simulink model "sampleModel282"  (R2021b)
settings: Solver=VariableStepAuto  StartTime=0.0  StopTime=10.0  RelTol=1e-3
undefined symbols (not defined in the file or in its folder): DiscIntNeverNeededParam, Newton, Raphson
libraries: simulink x13, slpidlib x2
settings Model: Creator=user  LastModifiedBy=user

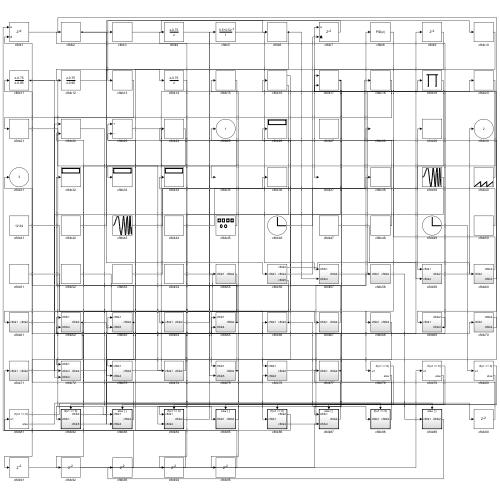
[thumbnail: Simulink's stored preview of the top-level diagram]
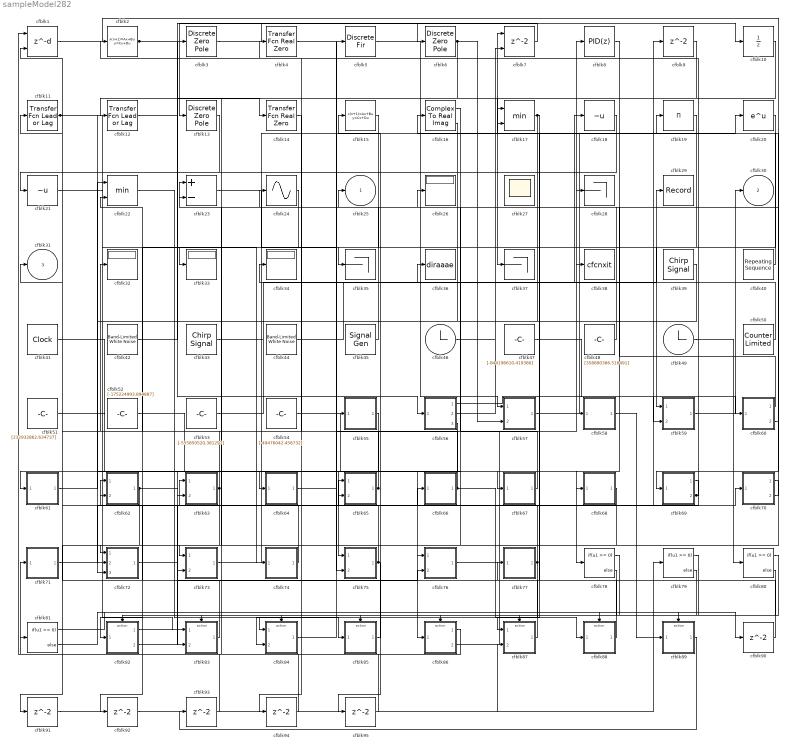
== system sampleModel282 ==
  cfblk1 : Delay  DelayLengthSource=Input port  SampleTime=1
      settings: InputPortMap=u0,p1
  cfblk10 : UnitDelay  HasFrameUpgradeWarning=on
  cfblk11 : simulink/Discrete/Transfer Fcn Lead or Lag  PoleZ=0.95  ZeroZ=0.75  ICPrevOutput=0.0  ICPrevInput=0.0  DoSatur=off
      settings: SourceProductBaseCode=SL
  cfblk12 : simulink/Discrete/Transfer Fcn Lead or Lag  PoleZ=0.95  ZeroZ=0.75  ICPrevOutput=0.0  ICPrevInput=0.0  DoSatur=off
      settings: SourceProductBaseCode=SL
  cfblk13 : DiscreteZeroPole  Poles=[0 0.5]  Gain=1
  cfblk14 : simulink/Discrete/Transfer Fcn Real Zero  ZeroZ=0.75  ICPrevInput=0.0  DoSatur=off
      settings: SourceProductBaseCode=SL
  cfblk15 : DiscreteStateSpace
  cfblk16 : ComplexToRealImag
  cfblk17 : MinMax  Inputs=2
  cfblk18 : UnaryMinus
  cfblk19 : Product  Inputs=*
  cfblk2 : DiscreteStateSpace
  cfblk20 : Math  SaturateOnIntegerOverflow=on
  cfblk21 : UnaryMinus
  cfblk22 : MinMax  Inputs=2
  cfblk23 : Sum  Inputs=+-
  cfblk24 : Sin  TimeSource=Use external signal  SampleTime=0
  cfblk{26,32..34} (4 alike) : Display
  cfblk27 : Scope
      settings: Floating=on
  cfblk28 : Terminator
  cfblk29 : Record  FileSettingsInternal="{\"entries\":[{\"content\":{\"excelSettings\":{\"content\":{},\"type\":\"Streamout.ExcelSettings\"}},\"type\":\"Streamout.FileSettingStorage\",\"uuid\":\"7d52aaf1-a181-40a9-9f35-a4ee466a9437\"}],\"packageUris\":[\"http://schema.mathworks.com/mf0/streamout_blocks/R2020a\"],\"version\":\"1.0\"}"  SignalsInternal="{\"entries\":[{\"content\":{\"signals\":[{\"content\":{\"blockPath\":[\"sampleModel282/cfblk29\"],\"channel\":[],\"dimensions\":[1],\"domain\":\"sampleModel282/cfblk29\",\"lineColor\":\"#fe330a\",\"plots\":[1],\"port\":1,\"sid\":[\"\"],\"signalID\":12055,\"signalName\":\"cfblk44\"},\"type\":\"RecordBlkView.Signal\",\"uuid\":\"b13949a6-b872-4204-8168-bd2ff3b91c96\"}]},\"type\":\"RecordBlkView.InputSignals\",\"uuid\":\"624ad5e0-89e9-4b40-8b6d-38fdad05cf61\"}],\"packageUris\":[\"http://schema.mathworks.com/mf0/streamout_blocks/R2020a\"],\"version\":\"1.0\"}"  VisualizationBindings="{\"sparklinesplugin\":{\"info\":[{\"bindingParametersList\":[],\"subplotID\":1}]}}"
  cfblk3 : DiscreteZeroPole  Poles=[0 0.5]  Gain=1
  cfblk35 : Terminator
  cfblk36 : ToWorkspace  VariableName=diraaae  SaveFormat=Timeseries  SampleTime=-1
  cfblk37 : Terminator
  cfblk38 : ToWorkspace  VariableName=cfcnxit  SaveFormat=Timeseries  SampleTime=-1
  cfblk39 : simulink/Sources/Chirp Signal  f1=[-918796217.277250]  T=[209630549.762623]  f2=[869455804.369112]
  cfblk4 : simulink/Discrete/Transfer Fcn Real Zero  ZeroZ=0.75  ICPrevInput=0.0  DoSatur=off
      settings: SourceProductBaseCode=SL
  cfblk40 : simulink/Sources/Repeating Sequence  rep_seq_t=[0 2]  rep_seq_y=[-594596007.538170, -429150568.442471]
  cfblk41 : DigitalClock
  cfblk42 : simulink/Sources/Band-Limited White Noise  Cov=[4229171843.958756]  Ts=0.1  seed=[8757087185.000000]
  cfblk43 : simulink/Sources/Chirp Signal  f1=[-499823119.966039]  T=[264408272.030996]  f2=[-997298266.489782]
  cfblk44 : simulink/Sources/Band-Limited White Noise  Cov=[7984496072.470979]  Ts=0.1  seed=[8150561720.000000]
  cfblk45 : SignalGenerator  Amplitude=[-24924778.301596]  Units=rad/sec
  cfblk46 : Clock
  cfblk47 : Constant  Value=[-844196610.419380]  SampleTime=1
  cfblk48 : Constant  Value=[358890386.516491]  SampleTime=1
  cfblk49 : Clock
  cfblk5 : DiscreteFir  SampleTime=1
  cfblk50 : simulink/Sources/Counter Limited  uplimit=[119.000000]  tsamp=-1
  cfblk51 : Constant  Value=[232932862.634737]  SampleTime=1
  cfblk52 : Constant  Value=[-175224993.894887]  SampleTime=1
  cfblk53 : Constant  Value=[-555850520.381297]  SampleTime=1
  cfblk54 : Constant  Value=[-49476042.458732]  SampleTime=1
  cfblk55 : Subsystem
  cfblk56 : Subsystem
  cfblk57 : Subsystem
  cfblk58 : Subsystem
  cfblk59 : Subsystem
  cfblk6 : DiscreteZeroPole  Poles=[0 0.5]  Gain=1
  cfblk60 : Subsystem
  cfblk61 : Subsystem
  cfblk62 : Subsystem
  cfblk63 : Subsystem
  cfblk64 : Subsystem
  cfblk65 : Subsystem
  cfblk66 : Subsystem
  cfblk67 : Subsystem
  cfblk68 : Subsystem
  cfblk69 : Subsystem
  cfblk7 : Delay  ShowEnablePort=on  SampleTime=1
      settings: InputPortMap=u0,e6
  cfblk70 : Subsystem
  cfblk71 : Subsystem
  cfblk72 : Subsystem
  cfblk73 : Subsystem
  cfblk74 : Subsystem
  cfblk75 : Subsystem
  cfblk76 : Subsystem
  cfblk77 : Subsystem
  cfblk{78..81} (4 alike) : If  IfExpression=u1 >= 0  SampleTime=1
  cfblk8 : slpidlib/PID Controller  Controller=PID  Form=Parallel  TimeDomain=Discrete-time  UseExternalTs=off  SampleTime=1  IntegratorMethod=Forward Euler  FilterMethod=Forward Euler  ControllerParametersSource=internal  P=1  I=1  D=0  UseFilter=on  N=100  TunerSelectOption=Transfer Function Based (PID Tuner App)  InitialConditionSource=internal  InitialConditionForIntegrator=0  InitialConditionForFilter=0  DifferentiatorICPrevScaledInput=0  ExternalReset=none  TrackingMode=off  Kt=1  LimitOutput=off  SatLimitsSource=internal  UpperSaturationLimit=inf  LowerSaturationLimit=-inf  LinearizeAsGain=off  AntiWindupMode=none  Kb=1  POutMin=[]  POutMax=[]  IOutMin=[]  IOutMax=[]  DOutMin=[]  DOutMax=[]  NOutMin=[]  NOutMax=[]  SumOutMin=[]  SumOutMax=[]  SaturationOutMin=[]  SaturationOutMax=[]  PParamMin=[]  PParamMax=[]  IParamMin=[]  IParamMax=[]  DParamMin=[]  DParamMax=[]  NParamMin=[]  NParamMax=[]  KbParamMin=[]  KbParamMax=[]  KtParamMin=[]  KtParamMax=[]  KbOutMin=[]  KbOutMax=[]  KtOutMin=[]  KtOutMax=[]  IntegratorOutMin=[]  IntegratorOutMax=[]  FilterOutMin=[]  FilterOutMax=[]  SumI1OutMin=[]  SumI1OutMax=[]  SumI2OutMin=[]  SumI2OutMax=[]  SumI3OutMin=[]  SumI3OutMax=[]  SumI4OutMin=[]  SumI4OutMax=[]  SumDOutMin=[]  SumDOutMax=[]  DifferentiatorOutMin=[]  DifferentiatorOutMax=[]  FilterDiffOutCoefMin=[]  FilterDiffOutCoefMax=[]  ReciprocalOutMin=[]  ReciprocalOutMax=[]  SumDenOutMin=[]  SumDenOutMax=[]  SumNumOutMin=[]  SumNumOutMax=[]  DivideOutMin=[]  DivideOutMax=[]  UdiffTsProdOutMin=[]  UdiffTsProdOutMax=[]  NTsProdOutMin=[]  NTsProdOutMax=[]  UintegralTsProdOutMin=[]  UintegralTsProdOutMax=[]  UngainTsProdOutMin=[]  UngainTsProdOutMax=[]  IntegratorContinuousStateAttributes=''  IntegratorStateMustResolveToSignalObject=off  IntegratorRTWStateStorageClass=Auto  FilterContinuousStateAttributes=''  FilterStateMustResolveToSignalObject=off  FilterRTWStateStorageClass=Auto  ParallelPVariant=InternalParameters  IdealPVariant=Disabled  IVariant=InternalParameters  DVariant=InternalParameters  IntegratorVariant=Discrete  SatVariant=Disabled  AWVariant=Passthrough  PCopyVariant=Disabled  TRVariant=Disabled  FdbkBlocksVariant=Forward  IdealPFdbkVariant=Disabled  SatFdbkVariant=Disabled  DerivativeFilterVariant=ForwardEulerFilter  NVariant=InternalParameters  NCopyVariant=Disabled  FilterICVariant=InternalICsFilter  IntegratorICVariant=InternalICs  ExternalResetVariant=Disabled  TRSumVariant=Passthrough  SumFdbkVariant=Disabled  SumVariant=Sum_PID  TsampFilterVariant=InternalTs  TsampNgainVariant=Passthrough  TsampIntegralVariant=Passthrough  ExternalSaturationOutDataTypeStr=Inherit: Same as second input
  cfblk82 : Subsystem  TreatAsAtomicUnit=on
  cfblk83 : Subsystem  TreatAsAtomicUnit=on
  cfblk84 : Subsystem  TreatAsAtomicUnit=on
  cfblk85 : Subsystem  TreatAsAtomicUnit=on
  cfblk86 : Subsystem  TreatAsAtomicUnit=on
  cfblk87 : Subsystem  TreatAsAtomicUnit=on
  cfblk88 : Subsystem  TreatAsAtomicUnit=on
  cfblk89 : Subsystem  TreatAsAtomicUnit=on
  cfblk{9,90..95} (7 alike) : Delay  SampleTime=1
  cfblk25 : Outport
  cfblk30 : Outport  Port=2
  cfblk31 : Outport  Port=3
  wires:
  cfblk48/1 -> cfblk23/1
  cfblk10/1 -> cfblk37/1
  cfblk22/1 -> cfblk85/1(cfblk1)
  cfblk84/1(cfblk2) -> cfblk5/1
  cfblk20/1 -> cfblk59/1(cfblk1)
  cfblk11/1 -> cfblk83/1(cfblk1), cfblk63/2(cfblk5)
  cfblk59/1(cfblk2) -> cfblk30/1
  cfblk7/1 -> cfblk13/1
  cfblk86/1(cfblk2) -> cfblk71/1(cfblk1)
  cfblk58/1(cfblk2) -> cfblk89/1(cfblk1)
  cfblk73/1(cfblk2) -> cfblk20/1
  cfblk47/1 -> cfblk60/1(cfblk1)
  cfblk41/1 -> cfblk75/1(cfblk1)
  cfblk62/1(cfblk2) -> cfblk72/1(cfblk1), cfblk90/1
  cfblk56/1(cfblk2) -> cfblk59/2(cfblk4)
  cfblk42/1 -> cfblk3/1
  cfblk16/1 -> cfblk61/1(cfblk1)
  cfblk5/1 -> cfblk57/1(cfblk1)
  cfblk2/1 -> cfblk56/1(cfblk1), cfblk6/1
  cfblk1/1 -> cfblk69/1(cfblk1)
  cfblk49/1 -> cfblk80/1
  cfblk63/1(cfblk2) -> cfblk32/1, cfblk91/1
  cfblk86/2(cfblk4) -> cfblk8/1
  cfblk18/1 -> cfblk21/1
  cfblk57/1(cfblk2) -> cfblk19/1
  cfblk55/1(cfblk2) -> cfblk82/1(cfblk1)
  cfblk13/1 -> cfblk72/2(cfblk3)
  cfblk24/1 -> cfblk33/1
  cfblk40/1 -> cfblk7/1
  cfblk46/1 -> cfblk7/2
  cfblk65/1(cfblk2) -> cfblk11/1, cfblk22/2
  cfblk52/1 -> cfblk78/1
  cfblk53/1 -> cfblk36/1
  cfblk85/1(cfblk2) -> cfblk15/1
  cfblk61/1(cfblk2) -> cfblk22/1
  cfblk77/1(cfblk2) -> cfblk65/1(cfblk1), cfblk84/2(cfblk4)
  cfblk51/1 -> cfblk86/1(cfblk1)
  cfblk15/1 -> cfblk35/1
  cfblk56/2(cfblk4) -> cfblk38/1
  cfblk83/1(cfblk2) -> cfblk62/1(cfblk1)
  cfblk68/1(cfblk2) -> cfblk83/2(cfblk4)
  cfblk17/1 -> cfblk76/1(cfblk1), cfblk87/1(cfblk1)
  cfblk45/1 -> cfblk25/1
  cfblk74/1(cfblk2) -> cfblk31/1
  cfblk8/1 -> cfblk68/1(cfblk1)
  cfblk16/2 -> cfblk72/3(cfblk4)
  cfblk50/1 -> cfblk34/1
  cfblk54/1 -> cfblk67/1(cfblk1)
  cfblk56/3(cfblk5) -> cfblk64/1(cfblk1)
  cfblk76/1(cfblk2) -> cfblk9/1
  cfblk3/1 -> cfblk10/1
  cfblk88/1(cfblk2) -> cfblk17/1
  cfblk43/1 -> cfblk18/1
  cfblk69/1(cfblk2) -> cfblk62/2(cfblk4)
  cfblk87/1(cfblk2) -> cfblk77/1(cfblk1)
  cfblk67/1(cfblk2) -> cfblk26/1
  cfblk75/1(cfblk2) -> cfblk63/1(cfblk1), cfblk95/1
  cfblk71/1(cfblk2) -> cfblk66/1(cfblk1)
  cfblk82/1(cfblk2) -> cfblk65/2(cfblk4)
  cfblk6/1 -> cfblk12/1, cfblk57/2(cfblk4)
  cfblk44/1 -> cfblk29/1
  cfblk21/1 -> cfblk74/1(cfblk1)
  cfblk9/1 -> cfblk73/1(cfblk1)
  cfblk60/1(cfblk2) -> cfblk28/1
  cfblk23/1 -> cfblk75/2(cfblk5)
  cfblk72/1(cfblk2) -> cfblk70/1(cfblk1)
  cfblk69/2(cfblk4) -> cfblk2/1, cfblk17/2
  cfblk64/1(cfblk2) -> cfblk58/1(cfblk1)
  cfblk82/2(cfblk5) -> cfblk76/2(cfblk3)
  cfblk4/1 -> cfblk55/1(cfblk1)
  cfblk66/1(cfblk2) -> cfblk88/1(cfblk1), cfblk4/1
  cfblk39/1 -> cfblk84/1(cfblk1)
  cfblk12/1 -> cfblk14/1
  cfblk60/2(cfblk3) -> cfblk16/1
  cfblk70/1(cfblk2) -> cfblk73/2(cfblk4)
  cfblk70/2(cfblk4) -> cfblk24/1
  cfblk78/1 -> cfblk82/Action
  cfblk78/2 -> cfblk83/Action
  cfblk79/1 -> cfblk84/Action
  cfblk79/2 -> cfblk85/Action
  cfblk80/1 -> cfblk86/Action
  cfblk80/2 -> cfblk87/Action
  cfblk81/1 -> cfblk88/Action
  cfblk81/2 -> cfblk89/Action
  cfblk90/1 -> cfblk1/2
  cfblk91/1 -> cfblk87/2(cfblk4)
  cfblk19/1 -> cfblk92/1
  cfblk92/1 -> cfblk79/1
  cfblk89/1(cfblk2) -> cfblk93/1
  cfblk93/1 -> cfblk81/1
  cfblk14/1 -> cfblk94/1
  cfblk94/1 -> cfblk1/1
  cfblk95/1 -> cfblk23/2

== system sampleModel282/cfblk55 ==
  cfblk1 : Inport
  cfblk3 : Squeeze
  cfblk2 : Outport
  wires:
  cfblk1/1 -> cfblk3/1
  cfblk3/1 -> cfblk2/1

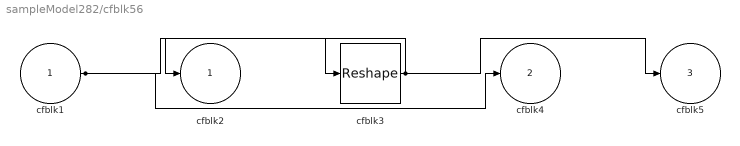
== system sampleModel282/cfblk56 ==
  cfblk1 : Inport
  cfblk3 : Reshape
  cfblk2 : Outport
  cfblk4 : Outport  Port=2
  cfblk5 : Outport  Port=3
  wires:
  cfblk3/1 -> cfblk2/1, cfblk5/1
  cfblk1/1 -> cfblk4/1, cfblk3/1

== system sampleModel282/cfblk57 ==
  cfblk1 : Inport
  cfblk4 : Inport  Port=2
  cfblk3 : DotProduct  InputSameDT=on  OutDataTypeStr=Inherit: Inherit via internal rule
  cfblk2 : Outport
  wires:
  cfblk4/1 -> cfblk2/1
  cfblk1/1 -> cfblk3/1, cfblk3/2

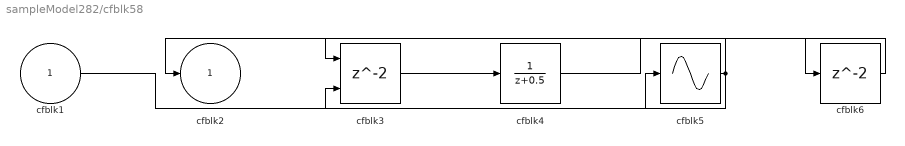
== system sampleModel282/cfblk58 ==
  cfblk1 : Inport
  cfblk3 : Delay  ShowEnablePort=on  SampleTime=1
      settings: InputPortMap=u0,e6
  cfblk4 : DiscreteTransferFcn  SampleTime=1
  cfblk5 : Sin  TimeSource=Use external signal  SampleTime=0
  cfblk6 : Delay  SampleTime=1
  cfblk2 : Outport
  wires:
  cfblk5/1 -> cfblk2/1, cfblk3/2
  cfblk1/1 -> cfblk5/1
  cfblk3/1 -> cfblk4/1
  cfblk4/1 -> cfblk6/1
  cfblk6/1 -> cfblk3/1

== system sampleModel282/cfblk59 ==
  cfblk1 : Inport
  cfblk4 : Inport  Port=2
  cfblk3 : Abs
  cfblk2 : Outport
  wires:
  cfblk1/1 -> cfblk2/1
  cfblk4/1 -> cfblk3/1

== system sampleModel282/cfblk60 ==
  cfblk1 : Inport
  cfblk2 : Outport
  cfblk3 : Outport  Port=2
  wires:
  cfblk1/1 -> cfblk2/1, cfblk3/1

== system sampleModel282/cfblk61 ==
  cfblk1 : Inport
  cfblk3 : slpidlib/PID Controller (2DOF)  Controller=PID  Form=Parallel  TimeDomain=Discrete-time  UseExternalTs=off  SampleTime=1  IntegratorMethod=Forward Euler  FilterMethod=Forward Euler  ControllerParametersSource=internal  P=1  I=1  D=0  UseFilter=on  N=100  b=1  c=1  TunerSelectOption=Transfer Function Based (PID Tuner App)  InitialConditionSource=internal  InitialConditionForIntegrator=0  InitialConditionForFilter=0  DifferentiatorICPrevScaledInput=0  ExternalReset=none  TrackingMode=off  Kt=1  LimitOutput=off  SatLimitsSource=internal  UpperSaturationLimit=inf  LowerSaturationLimit=-inf  LinearizeAsGain=off  AntiWindupMode=none  Kb=1  POutMin=[]  POutMax=[]  IOutMin=[]  IOutMax=[]  DOutMin=[]  DOutMax=[]  NOutMin=[]  NOutMax=[]  bOutMin=[]  bOutMax=[]  cOutMin=[]  cOutMax=[]  SumOutMin=[]  SumOutMax=[]  SaturationOutMin=[]  SaturationOutMax=[]  PParamMin=[]  PParamMax=[]  IParamMin=[]  IParamMax=[]  DParamMin=[]  DParamMax=[]  NParamMin=[]  NParamMax=[]  bParamMin=[]  bParamMax=[]  cParamMin=[]  cParamMax=[]  KbParamMin=[]  KbParamMax=[]  KtParamMin=[]  KtParamMax=[]  KbOutMin=[]  KbOutMax=[]  KtOutMin=[]  KtOutMax=[]  IntegratorOutMin=[]  IntegratorOutMax=[]  FilterOutMin=[]  FilterOutMax=[]  SumI1OutMin=[]  SumI1OutMax=[]  SumI2OutMin=[]  SumI2OutMax=[]  SumI3OutMin=[]  SumI3OutMax=[]  SumI4OutMin=[]  SumI4OutMax=[]  SumDOutMin=[]  SumDOutMax=[]  Sum1OutMin=[]  Sum1OutMax=[]  Sum2OutMin=[]  Sum2OutMax=[]  Sum3OutMin=[]  Sum3OutMax=[]  DifferentiatorOutMin=[]  DifferentiatorOutMax=[]  FilterDiffOutCoefMin=[]  FilterDiffOutCoefMax=[]  ReciprocalOutMin=[]  ReciprocalOutMax=[]  SumDenOutMin=[]  SumDenOutMax=[]  SumNumOutMin=[]  SumNumOutMax=[]  DivideOutMin=[]  DivideOutMax=[]  UdiffTsProdOutMin=[]  UdiffTsProdOutMax=[]  NTsProdOutMin=[]  NTsProdOutMax=[]  UintegralTsProdOutMin=[]  UintegralTsProdOutMax=[]  UngainTsProdOutMin=[]  UngainTsProdOutMax=[]  IntegratorContinuousStateAttributes=''  IntegratorStateMustResolveToSignalObject=off  IntegratorRTWStateStorageClass=Auto  FilterContinuousStateAttributes=''  FilterStateMustResolveToSignalObject=off  FilterRTWStateStorageClass=Auto  ParallelPVariant=InternalParameters  IdealPVariant=Disabled  IVariant=InternalParameters  DVariant=InternalParameters  bVariant=InternalParameters  cVariant=InternalParameters  IntegratorVariant=Discrete  SatVariant=Disabled  AWVariant=Passthrough  PCopyVariant=Disabled  TRVariant=Disabled  FdbkBlocksVariant=Forward  IdealPFdbkVariant=Disabled  SatFdbkVariant=Disabled  DerivativeFilterVariant=ForwardEulerFilter  NVariant=InternalParameters  NCopyVariant=Disabled  FilterICVariant=InternalICsFilter  IntegratorICVariant=InternalICs  ExternalResetVariant=Disabled  TRSumVariant=Passthrough  SumFdbkVariant=Disabled  SumVariant=Sum_PID  TsampFilterVariant=InternalTs  TsampNgainVariant=Passthrough  TsampIntegralVariant=Passthrough  ExternalSaturationOutDataTypeStr=Inherit: Same as second input
      settings: SourceProductBaseCode=SL
  cfblk2 : Outport
  wires:
  cfblk3/1 -> cfblk2/1
  cfblk1/1 -> cfblk3/1, cfblk3/2

== system sampleModel282/cfblk62 ==
  cfblk1 : Inport
  cfblk4 : Inport  Port=2
  cfblk3 : simulink/Discrete/Transfer Fcn Lead or Lag  PoleZ=0.95  ZeroZ=0.75  ICPrevOutput=0.0  ICPrevInput=0.0  DoSatur=off
      settings: SourceProductBaseCode=SL
  cfblk2 : Outport
  wires:
  cfblk1/1 -> cfblk3/1
  cfblk4/1 -> cfblk2/1

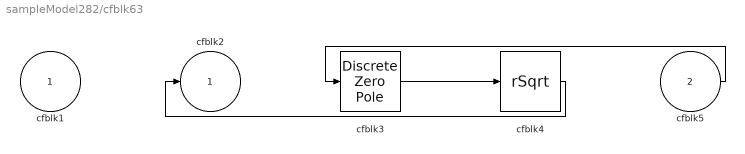
== system sampleModel282/cfblk63 ==
  cfblk1 : Inport
  cfblk5 : Inport  Port=2
  cfblk3 : DiscreteZeroPole  Poles=[0 0.5]  Gain=1
  cfblk4 : Sqrt  Operator=rSqrt  AlgorithmType=Newton-Raphson  SaturateOnIntegerOverflow=on
  cfblk2 : Outport
  wires:
  cfblk3/1 -> cfblk4/1
  cfblk5/1 -> cfblk3/1
  cfblk4/1 -> cfblk2/1

== system sampleModel282/cfblk64 ==
  cfblk1 : Inport
  cfblk3 : DiscreteZeroPole  Poles=[0 0.5]  Gain=1
  cfblk2 : Outport
  wires:
  cfblk3/1 -> cfblk2/1
  cfblk1/1 -> cfblk3/1

== system sampleModel282/cfblk65 ==
  cfblk1 : Inport
  cfblk4 : Inport  Port=2
  cfblk3 : Constant  Value=[-645215386.097908]  SampleTime=1
  cfblk2 : Outport
  wires:
  cfblk1/1 -> cfblk2/1

== system sampleModel282/cfblk66 ==
  cfblk1 : Inport
  cfblk3 : Sqrt  SaturateOnIntegerOverflow=on
  cfblk4 : Constant  Value=[-123973715.494942]  SampleTime=1
  cfblk2 : Outport
  wires:
  cfblk1/1 -> cfblk3/1
  cfblk4/1 -> cfblk2/1

== system sampleModel282/cfblk67 ==
  cfblk1 : Inport
  cfblk3 : Constant  Value=[387962848.922604]  SampleTime=1
  cfblk2 : Outport
  wires:
  cfblk1/1 -> cfblk2/1

== system sampleModel282/cfblk68 ==
  cfblk1 : Inport
  cfblk3 : ComplexToRealImag
  cfblk4 : ComplexToRealImag
  cfblk2 : Outport
  wires:
  cfblk4/1 -> cfblk3/1
  cfblk1/1 -> cfblk4/1
  cfblk4/2 -> cfblk2/1

== system sampleModel282/cfblk69 ==
  cfblk1 : Inport
  cfblk3 : Constant  Value=[-721714749.649663]  SampleTime=1
  cfblk2 : Outport
  cfblk4 : Outport  Port=2
  wires:
  cfblk1/1 -> cfblk4/1
  cfblk3/1 -> cfblk2/1

== system sampleModel282/cfblk70 ==
  cfblk1 : Inport
  cfblk3 : Product
  cfblk2 : Outport
  cfblk4 : Outport  Port=2
  wires:
  cfblk1/1 -> cfblk2/1, cfblk3/1, cfblk3/2
  cfblk3/1 -> cfblk4/1

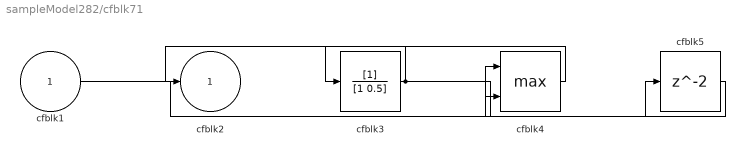
== system sampleModel282/cfblk71 ==
  cfblk1 : Inport
  cfblk3 : DiscreteFilter  SampleTime=1
  cfblk4 : MinMax  Function=max  Inputs=2
  cfblk5 : Delay  SampleTime=1
  cfblk2 : Outport
  wires:
  cfblk4/1 -> cfblk3/1
  cfblk1/1 -> cfblk4/1
  cfblk3/1 -> cfblk2/1, cfblk5/1
  cfblk5/1 -> cfblk4/2

== system sampleModel282/cfblk72 ==
  cfblk1 : Inport
  cfblk3 : Inport  Port=2
  cfblk4 : Inport  Port=3
  cfblk2 : Outport
  wires:
  cfblk4/1 -> cfblk2/1

== system sampleModel282/cfblk73 ==
  cfblk1 : Inport
  cfblk4 : Inport  Port=2
  cfblk3 : Product
  cfblk2 : Outport
  wires:
  cfblk3/1 -> cfblk2/1
  cfblk4/1 -> cfblk3/1
  cfblk1/1 -> cfblk3/2

== system sampleModel282/cfblk74 ==
  cfblk1 : Inport
  cfblk3 : DiscreteZeroPole  Poles=[0 0.5]  Gain=1
  cfblk2 : Outport
  wires:
  cfblk1/1 -> cfblk2/1, cfblk3/1

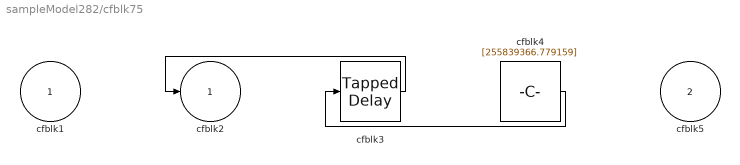
== system sampleModel282/cfblk75 ==
  cfblk1 : Inport
  cfblk5 : Inport  Port=2
  cfblk3 : simulink/Discrete/Tapped Delay  vinit=0.0  samptime=-1  NumDelays=1  DelayOrder=Oldest  includeCurrent=off
  cfblk4 : Constant  Value=[255839366.779159]  SampleTime=1
  cfblk2 : Outport
  wires:
  cfblk3/1 -> cfblk2/1
  cfblk4/1 -> cfblk3/1

== system sampleModel282/cfblk76 ==
  cfblk1 : Inport
  cfblk3 : Inport  Port=2
  cfblk2 : Outport
  wires:
  cfblk3/1 -> cfblk2/1

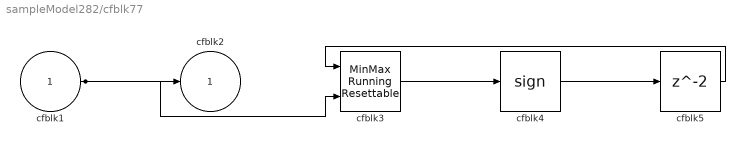
== system sampleModel282/cfblk77 ==
  cfblk1 : Inport
  cfblk3 : simulink/Math Operations/MinMax Running Resettable  Function=min  vinit=0.0
  cfblk4 : Signum
  cfblk5 : Delay  SampleTime=1
  cfblk2 : Outport
  wires:
  cfblk1/1 -> cfblk2/1, cfblk3/2
  cfblk3/1 -> cfblk4/1
  cfblk4/1 -> cfblk5/1
  cfblk5/1 -> cfblk3/1

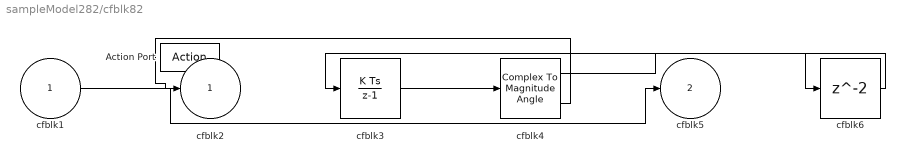
== system sampleModel282/cfblk82 ==
  cfblk1 : Inport
  Action Port : ActionPort  ActionPortLabel=if(u1 >= 0)
  cfblk3 : DiscreteIntegrator  SampleTime=-1  ICPrevOutput=DiscIntNeverNeededParam  ICPrevScaledInput=DiscIntNeverNeededParam
  cfblk4 : ComplexToMagnitudeAngle
  cfblk6 : Delay
  cfblk2 : Outport
  cfblk5 : Outport  Port=2
  wires:
  cfblk1/1 -> cfblk5/1
  cfblk3/1 -> cfblk4/1
  cfblk4/2 -> cfblk2/1
  cfblk4/1 -> cfblk6/1
  cfblk6/1 -> cfblk3/1

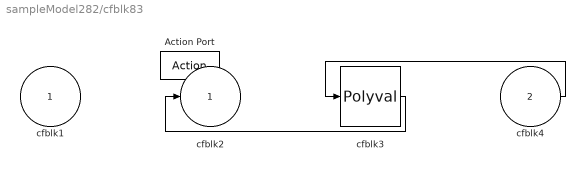
== system sampleModel282/cfblk83 ==
  cfblk1 : Inport
  cfblk4 : Inport  Port=2
  Action Port : ActionPort  ActionPortLabel=else
  cfblk3 : Polyval  Coefs=[ +2.081618890e-019, -1.441693666e-014, +4.719686976e-010, -8.536869453e-006, +1.621573104e-001, -8.087801117e+001 ]
  cfblk2 : Outport
  wires:
  cfblk4/1 -> cfblk3/1
  cfblk3/1 -> cfblk2/1

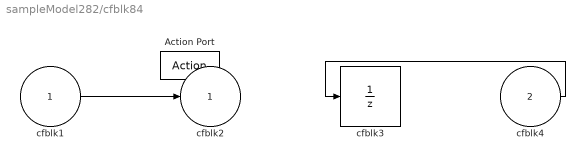
== system sampleModel282/cfblk84 ==
  cfblk1 : Inport
  cfblk4 : Inport  Port=2
  Action Port : ActionPort  ActionPortLabel=if(u1 >= 0)
  cfblk3 : UnitDelay  SampleTime=-1  HasFrameUpgradeWarning=on
  cfblk2 : Outport
  wires:
  cfblk1/1 -> cfblk2/1
  cfblk4/1 -> cfblk3/1

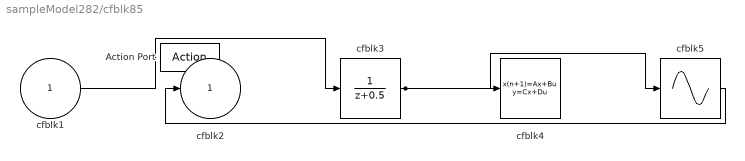
== system sampleModel282/cfblk85 ==
  cfblk1 : Inport
  Action Port : ActionPort  ActionPortLabel=else
  cfblk3 : DiscreteTransferFcn
  cfblk4 : DiscreteStateSpace  SampleTime=-1
  cfblk5 : Sin  TimeSource=Use external signal  SampleTime=0
  cfblk2 : Outport
  wires:
  cfblk5/1 -> cfblk2/1
  cfblk1/1 -> cfblk3/1
  cfblk3/1 -> cfblk5/1, cfblk4/1

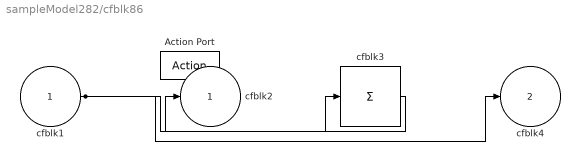
== system sampleModel282/cfblk86 ==
  cfblk1 : Inport
  Action Port : ActionPort  ActionPortLabel=if(u1 >= 0)
  cfblk3 : Sum  Inputs=+
  cfblk2 : Outport
  cfblk4 : Outport  Port=2
  wires:
  cfblk3/1 -> cfblk2/1
  cfblk1/1 -> cfblk4/1, cfblk3/1

== system sampleModel282/cfblk87 ==
  cfblk1 : Inport
  cfblk4 : Inport  Port=2
  Action Port : ActionPort  ActionPortLabel=else
  cfblk3 : Math  Operator=conj  SaturateOnIntegerOverflow=on
  cfblk2 : Outport
  wires:
  cfblk3/1 -> cfblk2/1
  cfblk1/1 -> cfblk3/1

== system sampleModel282/cfblk88 ==
  cfblk1 : Inport
  Action Port : ActionPort  ActionPortLabel=if(u1 >= 0)
  cfblk3 : DiscreteTransferFcn
  cfblk4 : ComplexToRealImag
  cfblk2 : Outport
  wires:
  cfblk3/1 -> cfblk2/1
  cfblk1/1 -> cfblk4/1
  cfblk4/1 -> cfblk3/1

== system sampleModel282/cfblk89 ==
  cfblk1 : Inport
  Action Port : ActionPort  ActionPortLabel=else
  cfblk3 : Sin  TimeSource=Use external signal  SampleTime=0
  cfblk2 : Outport
  wires:
  cfblk1/1 -> cfblk3/1
  cfblk3/1 -> cfblk2/1
